simulink model "Rc_circ"  (R2021a)
settings: Solver=VariableStepAuto  StartTime=0.0  StopTime=10.0  RelTol=1e-3
values from neighbouring files (symbols this model uses):
  C = 1e-6    (= 1e-06)    [RC_cir.m]
  R = 1000    [RC_cir.m]
  Vin = 5    [RC_cir.m]
settings Model: Creator=AHMED  LastModifiedBy=AHMED

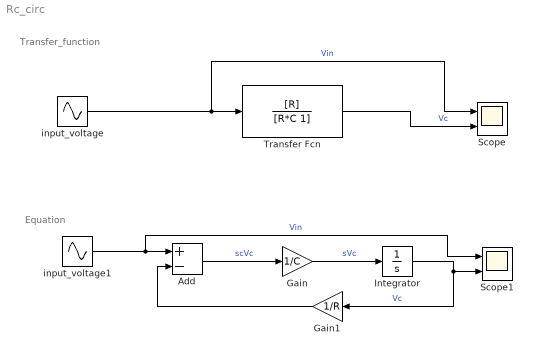
== system Rc_circ ==
  note: Equation
  note: Transfer_function
  Add : Sum  Inputs=+-
  Gain : Gain  Gain=1/C
  Gain1 : Gain  Gain=1/R
  Integrator : Integrator
  Scope : Scope  NumInputPorts=2
  Scope1 : Scope  NumInputPorts=2
  Transfer Fcn : TransferFcn  Numerator=[R]  Denominator=[R*C 1]
  input_voltage : Sin  Amplitude=Vin  Frequency=2*pi*2  SampleTime=0
  input_voltage1 : Sin  Amplitude=Vin  Frequency=2*pi*2  SampleTime=0
  wires:
  Transfer Fcn/1 -> Scope/2  "Vc"
  input_voltage/1 -> Scope/1, Transfer Fcn/1  "Vin"
  input_voltage1/1 -> Scope1/1, Add/1  "Vin"
  Add/1 -> Gain/1  "scVc"
  Gain/1 -> Integrator/1  "sVc"
  Integrator/1 -> Gain1/1, Scope1/2  "Vc"
  Gain1/1 -> Add/2
